simulink model "cv4_sp"  (R2019b)
settings: Solver=VariableStepAuto  StartTime=0.0  StopTime=6  RelTol=1e-3
values from neighbouring files (symbols this model uses):
  cp1 = 4186    [spoj.m]
  cp2 = 2420    [spoj.m]
  lambda12 = 1.02*10^6    (= 1020000)    [spoj.m]
  lambda2o = 2.1*10^4    (= 21000)    [spoj.m]
  M1 = 200    [spoj.m]
  M2 = 300    [spoj.m]
  S1 = 0.9817    [spoj.m]
  S2 = 1.4137    [spoj.m]
  T10 = 80    [spoj.m]
  T20 = 18    [spoj.m]
  To = 18    [spoj.m]
settings Model: Creator=student  LastModifiedBy=student

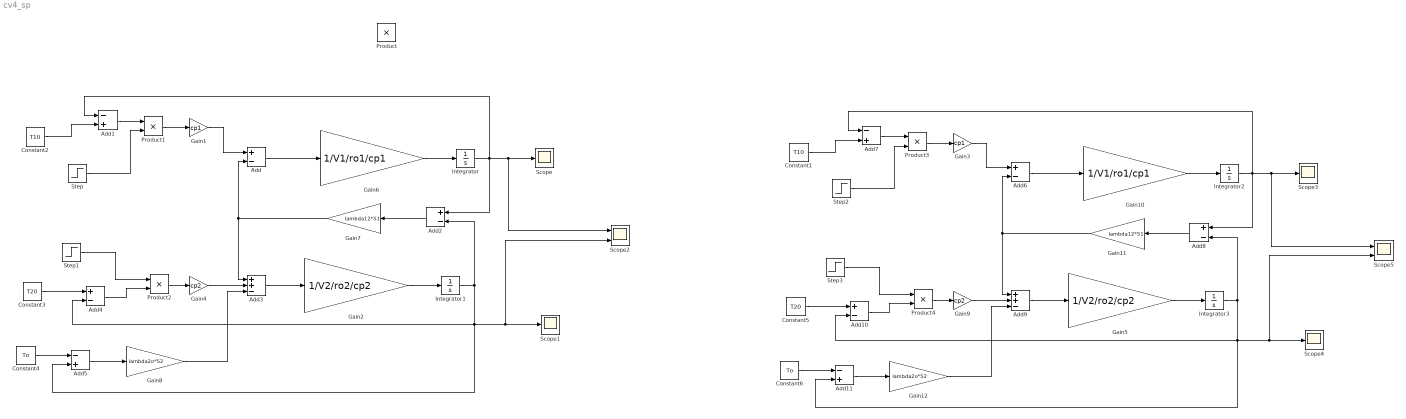
== system cv4_sp ==
  Add{,2,4,6,8,10} (6 alike) : Sum  Inputs=+-
  Add{1,5,7,11} (4 alike) : Sum  Inputs=-+
  Add3 : Sum  Inputs=++-
  Add9 : Sum  Inputs=++-
  Constant1 : Constant  Value=T10
  Constant2 : Constant  Value=T10
  Constant3 : Constant  Value=T20
  Constant4 : Constant  Value=To
  Constant5 : Constant  Value=T20
  Constant6 : Constant  Value=To
  Gain1 : Gain  Gain=cp1
  Gain10 : Gain  Gain=1/V1/ro1/cp1
  Gain11 : Gain  Gain=lambda12*S1
  Gain12 : Gain  Gain=lambda2o*S2
  Gain2 : Gain  Gain=1/V2/ro2/cp2
  Gain3 : Gain  Gain=cp1
  Gain4 : Gain  Gain=cp2
  Gain5 : Gain  Gain=1/V2/ro2/cp2
  Gain6 : Gain  Gain=1/V1/ro1/cp1
  Gain7 : Gain  Gain=lambda12*S1
  Gain8 : Gain  Gain=lambda2o*S2
  Gain9 : Gain  Gain=cp2
  Integrator : Integrator
  Integrator1 : Integrator
  Integrator2 : Integrator  InitialCondition=58.9
  Integrator3 : Integrator  InitialCondition=41.3
  Product{,1..4} (5 alike) : Product
  Scope{,1,3..4} (4 alike) : Scope
  Scope2 : Scope  NumInputPorts=2
  Scope5 : Scope  NumInputPorts=2
  Step : Step  Time=0  After=M1  SampleTime=0
  Step1 : Step  Time=0  After=M2  SampleTime=0
  Step2 : Step  Time=3  Before=M1  After=M1/2  SampleTime=0
  Step3 : Step  Time=0.5  Before=M2  After=M2/2  SampleTime=0
  wires:
  Gain1/1 -> Add/1
  Product1/1 -> Gain1/1
  Add1/1 -> Product1/1
  Integrator/1 -> Scope2/1, Scope/1, Add2/1, Add1/1
  Add2/1 -> Gain7/1
  Gain7/1 -> Add3/1, Add/2
  Add3/1 -> Gain2/1
  Gain4/1 -> Add3/2
  Product2/1 -> Gain4/1
  Step/1 -> Product1/2
  Step1/1 -> Product2/1
  Add4/1 -> Product2/2
  Integrator1/1 -> Add5/2, Scope2/2, Scope1/1, Add4/2, Add2/2
  Constant3/1 -> Add4/1
  Constant4/1 -> Add5/1
  Add5/1 -> Gain8/1
  Gain8/1 -> Add3/3
  Constant2/1 -> Add1/2
  Gain2/1 -> Integrator1/1
  Gain6/1 -> Integrator/1
  Add/1 -> Gain6/1
  Gain5/1 -> Integrator3/1
  Add9/1 -> Gain5/1
  Gain11/1 -> Add9/1, Add6/2
  Add8/1 -> Gain11/1
  Add6/1 -> Gain10/1
  Gain10/1 -> Integrator2/1
  Gain9/1 -> Add9/2
  Constant5/1 -> Add10/1
  Constant1/1 -> Add7/2
  Integrator3/1 -> Add11/2, Scope5/2, Scope4/1, Add10/2, Add8/2
  Gain3/1 -> Add6/1
  Step3/1 -> Product4/1
  Step2/1 -> Product3/2
  Product3/1 -> Gain3/1
  Add11/1 -> Gain12/1
  Add10/1 -> Product4/2
  Add7/1 -> Product3/1
  Product4/1 -> Gain9/1
  Integrator2/1 -> Scope5/1, Scope3/1, Add8/1, Add7/1
  Gain12/1 -> Add9/3
  Constant6/1 -> Add11/1
